simulink model "stateflow6DoF"  (R2024b)
settings: Solver=VariableStepAuto  StartTime=0.0  StopTime=inf  RelTol=1e-6
model workspace (MAT data in the model file):
  Apogee_stop = 0
  BG0 = [0.173648177667  0  -0.984807753012; 0  1  0; 0.984807753012  0  0.173648177667]
  e = 1.55334303427
  ignition_delay = 0
  include_turbulence = 1
  is_sustainer = 1
  launch_delay = 0
  q0 = [0.766044443119 0 0.642787609687 0]
  rocket = MultiStageRocket
  rocket.Name = "Argonia_2_19"
  rocket.stages(1) = Rocket
  rocket.stages(1).Name = "SustainerStage"
  rocket.stages(1).mass_dry = -2
  rocket.stages(1).XCG_dry = 1.653
  rocket.stages(1).MOI_dry = [0.005  0  0; 0  6.179  0; 0  0  6.179]
  rocket.stages(1).LREF = 0.059055
  rocket.stages(1).SREF = 0.0027390706167
  rocket.stages(1).NC_type = "KARMAN"
  rocket.stages(1).NC_length = 0.333375
  rocket.stages(1).NC_diam = 0.059055
  rocket.stages(1).AF1_length = 2.62509
  rocket.stages(1).AF1_diam = 0.059055
  rocket.stages(1).FN1_number = [3 3]
  rocket.stages(1).FN1_type = ["HEX" "HEX"]
  rocket.stages(1).FN1_NACA = ["" ""]
  rocket.stages(1).FN1_root = [0.2794 0.3556]
  rocket.stages(1).FN1_tip = [0.071628 0.071628]
  rocket.stages(1).FN1_height = [0.061214 0.0862076]
  rocket.stages(1).FN1_sweep = [72.6438266558 72.4181028235]
  rocket.stages(1).FN1_edgeRad = [0.000127 0.000127]
  rocket.stages(1).FN1_XLE = [1.497965 2.590165]
  rocket.stages(1).THICKNESS = [0.004064 0.004064]
  rocket.stages(1).ZUPPER = [0.00727272727273 0.00571428571429]
  rocket.stages(1).ZLOWER = [0.00727272727273 0.00571428571429]
  rocket.stages(1).LMAXU = [0.05 0.05]
  rocket.stages(1).LMAXL = [0.05 0.05]
  rocket.stages(1).LFLATU = [0.9 0.9]
  rocket.stages(1).LFLATL = [0.9 0.9]
  rocket.stages(1).m_table = [0.01  8.429; 0.02  8.423; 0.03  8.416; 0.04  8.409; 0.05  8.402; 0.06  8.396; 0.07  8.389; 0.08  8.383; 0.09  8.376; 0.1  8.369; 0.11  8.363; 0.12  8.356; 0.13  8.35; 0.14  8.343; 0.15  8.336; 0.16  8.33; 0.17  8.323; 0.18  8.317; 0.19  8.31; 0.2  8.304; 0.21  8.297; 0.22  8.291; 0.23  8.284; 0.24  8.278; 0.255  8.268; 0.278  8.253; 0.311  8.231; 0.361  8.199; 0.411  8.167; 0.461  8.135; 0.511  8.104; 0.561  8.072; 0.611  8.04; 0.661  8.009; 0.711  7.977; 0.761  7.946; 0.811  7.914; 0.861  7.883; 0.911  7.852; 0.961  7.821; 1.003  7.795; 1.04  7.772; 1.076  7.75; 1.113  7.727; 1.154  7.702; 1.204  7.672; 1.254  7.641; 1.304  7.612; 1.352  7.583; 1.385  7.564; 1.415  7.546; 1.445  7.528; 1.479  7.508; 1.525  7.481; 1.575  7.452; 1.625  7.423; 1.658  7.404; 1.687  7.388; 1.716  7.371; 1.749  7.352; 1.799  7.325; 1.849  7.297; 1.888  7.276; 1.917  7.26; 1.946  7.244; 1.982  7.225; 2.032  7.199; 2.082  7.174; 2.113  7.159; 2.143  7.146; 2.181  7.132; 2.231  7.115; 2.281  7.1; 2.314  7.092; 2.35  7.083; 2.4  7.072; 2.45  7.064; 2.49  7.058; 2.531  7.051; 2.581  7.044; 2.631  7.04; 2.676  7.037; 2.726  7.035; 2.776  7.033; 2.826  7.033; 2.876  7.032; 2.926  7.032; 2.976  7.031; 3  7.031]
  rocket.stages(1).COM_table = [0.01  1.817; 0.02  1.816; 0.03  1.816; 0.04  1.815; 0.05  1.814; 0.06  1.814; 0.07  1.813; 0.08  1.812; 0.09  1.812; 0.1  1.811; 0.11  1.81; 0.12  1.81; 0.13  1.809; 0.14  1.808; 0.15  1.808; 0.16  1.807; 0.17  1.806; 0.18  1.806; 0.19  1.805; 0.2  1.805; 0.21  1.804; 0.22  1.803; 0.23  1.803; 0.24  1.802; 0.255  1.801; 0.278  1.799; 0.311  1.797; 0.361  1.794; 0.411  1.791; 0.461  1.787; 0.511  1.784; 0.561  1.781; 0.611  1.777; 0.661  1.774; 0.711  1.77; 0.761  1.767; 0.811  1.763; 0.861  1.76; 0.911  1.756; 0.961  1.753; 1.003  1.75; 1.04  1.747; 1.076  1.745; 1.113  1.742; 1.154  1.739; 1.204  1.736; 1.254  1.732; 1.304  1.728; 1.352  1.725; 1.385  1.723; 1.415  1.721; 1.445  1.718; 1.479  1.716; 1.525  1.713; 1.575  1.709; 1.625  1.705; 1.658  1.703; 1.687  1.701; 1.716  1.699; 1.749  1.696; 1.799  1.693; 1.849  1.689; 1.888  1.686; 1.917  1.684; 1.946  1.682; 1.982  1.68; 2.032  1.676; 2.082  1.673; 2.113  1.671; 2.143  1.669; 2.181  1.667; 2.231  1.665; 2.281  1.663; 2.314  1.662; 2.35  1.66; 2.4  1.659; 2.45  1.658; 2.49  1.657; 2.531  1.656; 2.581  1.655; 2.631  1.654; 2.676  1.654; 2.726  1.654; 2.776  1.653; 2.826  1.653; 2.876  1.653; 2.926  1.653; 2.976  1.653; 3  1.653]
  rocket.stages(1).MOI_table = [0.006 0.006 0.006 0.006 0.006 0.006 0.006 0.006 0.006 0.006 0.006 0.006 ... (801 elements, 89x3x3)]
  rocket.stages(1).motor = SolidMotor
  rocket.stages(1).motor.Name = "AeroTech HP-L1000W"
  rocket.stages(1).motor.thrust_table = [0.01  332.093; 0.02  1267.419; 0.03  1294.701; 0.04  1313.086; 0.05  1319.183; 0.06  1312.991; 0.07  1306.8; 0.08  1300.608; 0.09  1294.416; 0.1  1288.224; 0.11  1282.033; 0.12  1275.841; 0.13  1269.649; 0.14  1263.457; 0.15  1257.266; 0.16  1251.074; 0.17  1244.882; 0.18  1238.69; 0.19  1232.499; 0.2  1228.068; 0.21  1234.206; 0.22  1242.105; 0.23  1250.004; 0.24  1257.903; 0.255  1266.148; 0.278  1259.177; 0.311  1245.662; 0.361  1247.95; 0.411  1239.736; 0.461  1217.022; 0.511  1219.715; 0.561  1222.613; 0.611  1225.365; 0.661  1224.251; 0.711  1221.415; 0.761  1218.579; 0.811  1215.428; 0.861  1210.092; 0.911  1204.338; 0.961  1198.584; 1.003  1193.301; 1.04  1188.756; 1.076  1184.609; 1.113  1181.332; 1.154  1178.132; 1.204  1174.387; 1.254  1170.286; 1.304  1164.499; 1.352  1156.078; 1.385  1149.076; 1.415  1143.601; 1.445  1138.375; 1.479  1132.822; 1.525  1125.967; 1.575  1118.328; 1.625  1110.52; 1.658  1103.994; 1.687  1099.14; 1.716  1094.669; 1.749  1089.82; 1.799  1079.006; 1.849  1063.36; 1.888  1051.16; 1.917  1048.821; 1.946  1047.63; 1.982  1046.301; 2.032  1026.685; 2.082  960.979; 2.113  897.673; 2.143  821.694; 2.181  741.135; 2.231  659.341; 2.281  569.943; 2.314  513.948; 2.35  472.863; 2.4  421.86; 2.45  364.372; 2.49  313.538; 2.531  267.801; 2.581  216.206; 2.631  165.618; 2.676  121.617; 2.726  80.868; 2.776  49.756; 2.826  35.45; 2.876  26.526; 2.926  17.603; 2.976  8.679; 3  2.109]
  rocket.stages(1).motor.mass_table = [0.01  3.984; 0.02  3.977; 0.03  3.971; 0.04  3.964; 0.05  3.957; 0.06  3.951; 0.07  3.944; 0.08  3.937; 0.09  3.931; 0.1  3.924; 0.11  3.918; 0.12  3.911; 0.13  3.904; 0.14  3.898; 0.15  3.891; 0.16  3.885; 0.17  3.878; 0.18  3.871; 0.19  3.865; 0.2  3.858; 0.21  3.852; 0.22  3.845; 0.23  3.839; 0.24  3.832; 0.255  3.823; 0.278  3.808; 0.311  3.786; 0.361  3.754; 0.411  3.722; 0.461  3.69; 0.511  3.659; 0.561  3.627; 0.611  3.595; 0.661  3.564; 0.711  3.532; 0.761  3.5; 0.811  3.469; 0.861  3.438; 0.911  3.407; 0.961  3.376; 1.003  3.35; 1.04  3.327; 1.076  3.305; 1.113  3.282; 1.154  3.257; 1.204  3.227; 1.254  3.196; 1.304  3.166; 1.352  3.138; 1.385  3.118; 1.415  3.101; 1.445  3.083; 1.479  3.063; 1.525  3.036; 1.575  3.007; 1.625  2.978; 1.658  2.959; 1.687  2.943; 1.716  2.926; 1.749  2.907; 1.799  2.88; 1.849  2.852; 1.888  2.83; 1.917  2.815; 1.946  2.799; 1.982  2.779; 2.032  2.754; 2.082  2.728; 2.113  2.714; 2.143  2.701; 2.181  2.687; 2.231  2.67; 2.281  2.655; 2.314  2.647; 2.35  2.638; 2.4  2.626; 2.45  2.619; 2.49  2.612; 2.531  2.606; 2.581  2.599; 2.631  2.595; 2.676  2.592; 2.726  2.589; 2.776  2.588; 2.826  2.588; 2.876  2.587; 2.926  2.587; 2.976  2.586; 3  2.586]
  rocket.stages(1).motor.dry_mass = 2.586
  rocket.stages(1).motor.total_prop_mass = 1.398
  rocket.stages(1).motor.motor_length = 0.635
  rocket.stages(1).motor.motor_diameter = 0.054
  rocket.stages(2) = Rocket
  rocket.stages(2).Name = "Stage"
  rocket.stages(2).mass_dry = -1
  rocket.stages(2).XCG_dry = 0.659935
  rocket.stages(2).MOI_dry = [0.002  0  0; 0  0.252  0; 0  0  0.252]
  rocket.stages(2).LREF = 0.059055
  rocket.stages(2).SREF = 0.0027390706167
  rocket.stages(2).NC_diam = 0.059055
  rocket.stages(2).AF1_length = 1.1684
  rocket.stages(2).AF1_diam = 0.059055
  rocket.stages(2).FN1_number = 3
  rocket.stages(2).FN1_root = 0.3556
  rocket.stages(2).FN1_tip = 0.071628
  rocket.stages(2).FN1_height = 0.0862076
  rocket.stages(2).FN1_sweep = 72.4181028235
  rocket.stages(2).FN1_XLE = 0.8001
  rocket.stages(2).THICKNESS = 0.004064
  rocket.stages(2).ZUPPER = 0.00571428571429
  rocket.stages(2).ZLOWER = 0.00571428571429
  rocket.stages(2).LMAXU = 0.05
  rocket.stages(2).LMAXL = 0.05
  rocket.stages(2).LFLATU = 0.9
  rocket.stages(2).LFLATL = 0.9
  rocket.stages(2).m_table = [8.022  2.518; 8.055  2.518]
  rocket.stages(2).COM_table = [6.231935  0.659935; 6.264935  0.659935]
  rocket.stages(2).MOI_table = reshape([0.002 0.002 0 0 0 0 0 0 0.252 0.252 0 0 0 0 0 0 0.252 0.252], [2 3 3])
  rocket.stages(2).motor = SolidMotor
  rocket.stages(2).motor.Name = "AeroTech HP-L1000W"
  rocket.stages(2).motor.thrust_table = [0.01  332.093; 0.02  1267.419; 0.03  1294.701; 0.04  1313.086; 0.05  1319.183; 0.06  1312.991; 0.07  1306.8; 0.08  1300.608; 0.09  1294.416; 0.1  1288.224; 0.11  1282.033; 0.12  1275.841; 0.13  1269.649; 0.14  1263.457; 0.15  1257.266; 0.16  1251.074; 0.17  1244.882; 0.18  1238.69; 0.19  1232.499; 0.2  1228.068; 0.21  1234.206; 0.22  1242.105; 0.23  1250.004; 0.24  1257.903; 0.255  1266.148; 0.278  1259.177; 0.311  1245.662; 0.361  1247.95; 0.411  1239.736; 0.461  1217.022; 0.511  1219.715; 0.561  1222.613; 0.611  1225.365; 0.661  1224.251; 0.711  1221.415; 0.761  1218.579; 0.811  1215.428; 0.861  1210.092; 0.911  1204.338; 0.961  1198.584; 1.003  1193.301; 1.04  1188.756; 1.076  1184.609; 1.113  1181.332; 1.154  1178.132; 1.204  1174.387; 1.254  1170.286; 1.304  1164.499; 1.352  1156.078; 1.385  1149.076; 1.415  1143.601; 1.445  1138.375; 1.479  1132.822; 1.525  1125.967; 1.575  1118.328; 1.625  1110.52; 1.658  1103.994; 1.687  1099.14; 1.716  1094.669; 1.749  1089.82; 1.799  1079.006; 1.849  1063.36; 1.888  1051.16; 1.917  1048.821; 1.946  1047.63; 1.982  1046.301; 2.032  1026.685; 2.082  960.979; 2.113  897.673; 2.143  821.694; 2.181  741.135; 2.231  659.341; 2.281  569.943; 2.314  513.948; 2.35  472.863; 2.4  421.86; 2.45  364.372; 2.49  313.538; 2.531  267.801; 2.581  216.206; 2.631  165.618; 2.676  121.617; 2.726  80.868; 2.776  49.756; 2.826  35.45; 2.876  26.526; 2.926  17.603; 2.976  8.679; 3  2.109]
  rocket.stages(2).motor.mass_table = [0.01  3.984; 0.02  3.977; 0.03  3.971; 0.04  3.964; 0.05  3.957; 0.06  3.951; 0.07  3.944; 0.08  3.937; 0.09  3.931; 0.1  3.924; 0.11  3.918; 0.12  3.911; 0.13  3.904; 0.14  3.898; 0.15  3.891; 0.16  3.885; 0.17  3.878; 0.18  3.871; 0.19  3.865; 0.2  3.858; 0.21  3.852; 0.22  3.845; 0.23  3.839; 0.24  3.832; 0.255  3.823; 0.278  3.808; 0.311  3.786; 0.361  3.754; 0.411  3.722; 0.461  3.69; 0.511  3.659; 0.561  3.627; 0.611  3.595; 0.661  3.564; 0.711  3.532; 0.761  3.5; 0.811  3.469; 0.861  3.438; 0.911  3.407; 0.961  3.376; 1.003  3.35; 1.04  3.327; 1.076  3.305; 1.113  3.282; 1.154  3.257; 1.204  3.227; 1.254  3.196; 1.304  3.166; 1.352  3.138; 1.385  3.118; 1.415  3.101; 1.445  3.083; 1.479  3.063; 1.525  3.036; 1.575  3.007; 1.625  2.978; 1.658  2.959; 1.687  2.943; 1.716  2.926; 1.749  2.907; 1.799  2.88; 1.849  2.852; 1.888  2.83; 1.917  2.815; 1.946  2.799; 1.982  2.779; 2.032  2.754; 2.082  2.728; 2.113  2.714; 2.143  2.701; 2.181  2.687; 2.231  2.67; 2.281  2.655; 2.314  2.647; 2.35  2.638; 2.4  2.626; 2.45  2.619; 2.49  2.612; 2.531  2.606; 2.581  2.599; 2.631  2.595; 2.676  2.592; 2.726  2.589; 2.776  2.588; 2.826  2.588; 2.876  2.587; 2.926  2.587; 2.976  2.586; 3  2.586]
  rocket.stages(2).motor.dry_mass = 2.586
  rocket.stages(2).motor.total_prop_mass = 1.398
  rocket.stages(2).motor.motor_length = 0.635
  rocket.stages(2).motor.motor_diameter = 0.054
  rocket.stages(3) = Rocket
  rocket.stages(3).Name = "Sustainer"
  rocket.stages(3).mass_dry = -1
  rocket.stages(3).XCG_dry = 1.099
  rocket.stages(3).MOI_dry = [0.002  0  0; 0  0.967  0; 0  0  0.967]
  rocket.stages(3).LREF = 0.059055
  rocket.stages(3).SREF = 0.0027390706167
  rocket.stages(3).NC_type = "KARMAN"
  rocket.stages(3).NC_length = 0.333375
  rocket.stages(3).NC_diam = 0.059055
  rocket.stages(3).AF1_length = 1.45669
  rocket.stages(3).AF1_diam = 0.059055
  rocket.stages(3).FN1_number = 3
  rocket.stages(3).FN1_root = 0.2794
  rocket.stages(3).FN1_tip = 0.071628
  rocket.stages(3).FN1_height = 0.061214
  rocket.stages(3).FN1_sweep = 72.6438266558
  rocket.stages(3).FN1_XLE = 1.497965
  rocket.stages(3).THICKNESS = 0.004064
  rocket.stages(3).ZUPPER = 0.00727272727273
  rocket.stages(3).ZLOWER = 0.00727272727273
  rocket.stages(3).LMAXU = 0.05
  rocket.stages(3).LMAXL = 0.05
  rocket.stages(3).LFLATU = 0.9
  rocket.stages(3).LFLATL = 0.9
  rocket.stages(3).m_table = [0  7.031; 0.022  4.508; 0.055  4.496; 0.104  4.476; 0.154  4.46; 0.204  4.448; 0.254  4.436; 0.304  4.426; 0.354  4.416; 0.404  4.406; 0.454  4.396; 0.504  4.386; 0.554  4.377; 0.604  4.368; 0.654  4.359; 0.704  4.35; 0.754  4.341; 0.804  4.332; 0.854  4.323; 0.904  4.314; 0.954  4.305; 1.004  4.297; 1.054  4.288; 1.104  4.279; 1.154  4.271; 1.204  4.262; 1.254  4.253; 1.304  4.245; 1.354  4.236; 1.404  4.228; 1.454  4.219; 1.504  4.21; 1.554  4.202; 1.604  4.193; 1.654  4.185; 1.704  4.177; 1.754  4.168; 1.804  4.16; 1.854  4.152; 1.904  4.143; 1.954  4.135; 2.004  4.126; 2.054  4.118; 2.104  4.109; 2.154  4.101; 2.204  4.093; 2.254  4.084; 2.304  4.076; 2.354  4.067; 2.404  4.059; 2.454  4.05; 2.504  4.042; 2.554  4.034; 2.604  4.025; 2.654  4.017; 2.704  4.008; 2.754  4; 2.804  3.992; 2.854  3.983; 2.904  3.975; 2.954  3.966; 3.004  3.958; 3.054  3.95; 3.104  3.942; 3.154  3.933; 3.204  3.925; 3.254  3.917; 3.304  3.909; 3.354  3.901; 3.404  3.893; 3.454  3.884; 3.504  3.876; 3.554  3.869; 3.604  3.861; 3.654  3.854; 3.704  3.846; 3.754  3.839; 3.804  3.831; 3.854  3.824; 3.904  3.816; 3.954  3.809; 4.004  3.801; 4.054  3.794; 4.104  3.788; 4.154  3.781; 4.204  3.775; 4.254  3.768; 4.304  3.761; 4.354  3.755; 4.404  3.748; 4.454  3.742; 4.504  3.735; 4.554  3.729; 4.604  3.723; 4.654  3.718; 4.704  3.712; 4.754  3.706; 4.804  3.7; 4.854  3.695; 4.904  3.689; 4.954  3.683; 5.004  3.678; 5.054  3.673; 5.104  3.668; 5.154  3.663; 5.204  3.659; 5.254  3.654; 5.304  3.649; 5.354  3.645; 5.404  3.64; 5.454  3.635; 5.504  3.631; 5.554  3.627; 5.604  3.623; 5.654  3.62; 5.704  3.616; 5.754  3.612; 5.804  3.609; 5.854  3.605; 5.904  3.601; 5.954  3.598; 6.004  3.594; 6.054  3.592; 6.104  3.589; 6.154  3.587; 6.204  3.584; 6.254  3.582; 6.304  3.579; 6.354  3.577; 6.404  3.574; 6.454  3.572; 6.504  3.569; 6.554  3.568; 6.604  3.568; 6.654  3.567; 6.704  3.566; 6.754  3.565; 6.804  3.564; 6.854  3.563; 6.904  3.562; 6.954  3.562; 7  3.561]
  rocket.stages(3).COM_table = [0  1.653; 0.022  1.208; 0.055  1.207; 0.104  1.205; 0.154  1.203; 0.204  1.202; 0.254  1.201; 0.304  1.2; 0.354  1.199; 0.404  1.198; 0.454  1.197; 0.504  1.197; 0.554  1.196; 0.604  1.195; 0.654  1.194; 0.704  1.193; 0.754  1.192; 0.804  1.191; 0.854  1.19; 0.904  1.19; 0.954  1.189; 1.004  1.188; 1.054  1.187; 1.104  1.186; 1.154  1.185; 1.204  1.184; 1.254  1.183; 1.304  1.183; 1.354  1.182; 1.404  1.181; 1.454  1.18; 1.504  1.179; 1.554  1.178; 1.604  1.177; 1.654  1.176; 1.704  1.175; 1.754  1.175; 1.804  1.174; 1.854  1.173; 1.904  1.172; 1.954  1.171; 2.004  1.17; 2.054  1.169; 2.104  1.168; 2.154  1.167; 2.204  1.166; 2.254  1.165; 2.304  1.165; 2.354  1.164; 2.404  1.163; 2.454  1.162; 2.504  1.161; 2.554  1.16; 2.604  1.159; 2.654  1.158; 2.704  1.157; 2.754  1.156; 2.804  1.155; 2.854  1.154; 2.904  1.153; 2.954  1.152; 3.004  1.151; 3.054  1.15; 3.104  1.149; 3.154  1.148; 3.204  1.147; 3.254  1.146; 3.304  1.145; 3.354  1.144; 3.404  1.143; 3.454  1.142; 3.504  1.141; 3.554  1.14; 3.604  1.139; 3.654  1.139; 3.704  1.138; 3.754  1.137; 3.804  1.136; 3.854  1.135; 3.904  1.134; 3.954  1.133; 4.004  1.132; 4.054  1.131; 4.104  1.13; 4.154  1.129; 4.204  1.129; 4.254  1.128; 4.304  1.127; 4.354  1.126; 4.404  1.125; 4.454  1.124; 4.504  1.123; 4.554  1.123; 4.604  1.122; 4.654  1.121; 4.704  1.12; 4.754  1.12; 4.804  1.119; 4.854  1.118; 4.904  1.117; 4.954  1.116; 5.004  1.116; 5.054  1.115; 5.104  1.114; 5.154  1.114; 5.204  1.113; 5.254  1.112; 5.304  1.112; 5.354  1.111; 5.404  1.11; 5.454  1.11; 5.504  1.109; 5.554  1.109; 5.604  1.108; 5.654  1.108; 5.704  1.107; 5.754  1.107; 5.804  1.106; 5.854  1.106; 5.904  1.105; 5.954  1.105; 6.004  1.104; 6.054  1.104; 6.104  1.103; 6.154  1.103; 6.204  1.103; 6.254  1.102; 6.304  1.102; 6.354  1.102; 6.404  1.101; 6.454  1.101; 6.504  1.1; 6.554  1.1; 6.604  1.1; 6.654  1.1; 6.704  1.1; 6.754  1.1; 6.804  1.1; 6.854  1.1; 6.904  1.099; 6.954  1.099; 7  1.099]
  rocket.stages(3).MOI_table = [0.005 0.003 0.003 0.003 0.003 0.003 0.003 0.003 0.003 0.003 0.003 0.003 ... (1278 elements, 142x3x3)]
  rocket.stages(3).motor = SolidMotor
  rocket.stages(3).motor.Name = "Loki Research K250-LW"
  rocket.stages(3).motor.thrust_table = [0 0.022 0.055 0.104 0.154 0.204 0.254 0.304 0.354 0.404 0.454 0.504 ... (284 elements, 142x2)]
  rocket.stages(3).motor.mass_table = [0  2.586; 0.022  1.787; 0.055  1.775; 0.104  1.754; 0.154  1.739; 0.204  1.726; 0.254  1.715; 0.304  1.705; 0.354  1.694; 0.404  1.684; 0.454  1.674; 0.504  1.665; 0.554  1.655; 0.604  1.646; 0.654  1.637; 0.704  1.628; 0.754  1.619; 0.804  1.611; 0.854  1.602; 0.904  1.593; 0.954  1.584; 1.004  1.575; 1.054  1.566; 1.104  1.558; 1.154  1.549; 1.204  1.54; 1.254  1.532; 1.304  1.523; 1.354  1.515; 1.404  1.506; 1.454  1.497; 1.504  1.489; 1.554  1.48; 1.604  1.472; 1.654  1.464; 1.704  1.455; 1.754  1.447; 1.804  1.438; 1.854  1.43; 1.904  1.422; 1.954  1.413; 2.004  1.405; 2.054  1.396; 2.104  1.388; 2.154  1.379; 2.204  1.371; 2.254  1.363; 2.304  1.354; 2.354  1.346; 2.404  1.337; 2.454  1.329; 2.504  1.32; 2.554  1.312; 2.604  1.304; 2.654  1.295; 2.704  1.287; 2.754  1.278; 2.804  1.27; 2.854  1.262; 2.904  1.253; 2.954  1.245; 3.004  1.236; 3.054  1.228; 3.104  1.22; 3.154  1.212; 3.204  1.204; 3.254  1.196; 3.304  1.187; 3.354  1.179; 3.404  1.171; 3.454  1.163; 3.504  1.155; 3.554  1.147; 3.604  1.14; 3.654  1.132; 3.704  1.125; 3.754  1.117; 3.804  1.11; 3.854  1.102; 3.904  1.094; 3.954  1.087; 4.004  1.079; 4.054  1.073; 4.104  1.066; 4.154  1.06; 4.204  1.053; 4.254  1.046; 4.304  1.04; 4.354  1.033; 4.404  1.027; 4.454  1.02; 4.504  1.013; 4.554  1.008; 4.604  1.002; 4.654  0.996; 4.704  0.99; 4.754  0.985; 4.804  0.979; 4.854  0.973; 4.904  0.967; 4.954  0.962; 5.004  0.956; 5.054  0.951; 5.104  0.947; 5.154  0.942; 5.204  0.937; 5.254  0.932; 5.304  0.928; 5.354  0.923; 5.404  0.918; 5.454  0.914; 5.504  0.909; 5.554  0.905; 5.604  0.902; 5.654  0.898; 5.704  0.894; 5.754  0.891; 5.804  0.887; 5.854  0.883; 5.904  0.88; 5.954  0.876; 6.004  0.872; 6.054  0.87; 6.104  0.867; 6.154  0.865; 6.204  0.863; 6.254  0.86; 6.304  0.858; 6.354  0.855; 6.404  0.853; 6.454  0.85; 6.504  0.848; 6.554  0.847; 6.604  0.846; 6.654  0.845; 6.704  0.844; 6.754  0.843; 6.804  0.843; 6.854  0.842; 6.904  0.841; 6.954  0.84; 7  0.839]
  rocket.stages(3).motor.dry_mass = 0.839
  rocket.stages(3).motor.total_prop_mass = 1.747
  rocket.stages(3).motor.motor_length = 0.499
  rocket.stages(3).motor.motor_diameter = 0.054
  second_ignition_stop = 0
  separation_delay = 5
  vertical_angle_lockout = 25
  wind_direction_table = [0  180; 1  180]
  wind_model_type = "Wind_Table"
  wind_speed_table = [0  7.15; 1  7.15]
values from neighbouring files (symbols this model uses):
  g = 9.81    [initialize_6DoF.m]
  latlong0 = [initial_conditions.lambda0, initial_conditions.mu0]    [initialize_6DoF.m]    (also in rail_output_to_6DoF_initial_conditions.m = deg2rad([launch_site.latitude;                      launch_s)
  v0_NED = GB0*initial_conditions.uvw0_B    [initialize_6DoF.m]
undefined symbols (not defined in the file or in its folder): aerotables, Cd, ChartModeType, deltat, FlightPhase2, HG0, l, launch_elevation, magnitude, mu, rho, S, uvw0_B
libraries: simulink_extras x6, aerolibfltsims x2, aerolibatmos2 x1, sharedtransform x1, aerolibanim x1
settings Model: DataDictionary=CombinedModelDictionary.sldd  Creator=thatf  LastModifiedBy=thatf
settings SolverCC: ZeroCrossAlgorithm=Adaptive
settings DebuggingCC: IgnoredZcDiagnostic=none
settings HardwareCC: ProdBitPerLong=64  ProdHWDeviceType=Intel->x86-64 (Linux 64)
settings SFSimCC: SimCustomHeaderCode=|
  | #include "pressure_altitude.h"
  | #include "flight_estimation.h"
  | #include "data.h"
  | #include "max_m10s.h"
  | #include "i2c/i2c.h"
settings SFSimCC: SimUserSources=|
  | Ccode/pressure_altitude.c
  | Ccode/my_func.c
  | Ccode/flight_estimation.c
  | Ccode/accel_est.c
  | Ccode/vector.c
settings RTWCC: Description=Simulink Desktop Real-Time  SystemTargetFile=sldrt.tlc  TemplateMakefile=sldrt.tmf  RTWCompilerOptimization=on
settings CodeAppCC: MaxIdLength=95
settings SimulinkDesktopRealTimeCC: TargetLibSuffix=_sldrt.a  TargetPreCompLibLocation=C:\Program Files\MATLAB\R2024b\toolbox\sldrt\lib\win64  ParMdlRefBuildCompliant=on

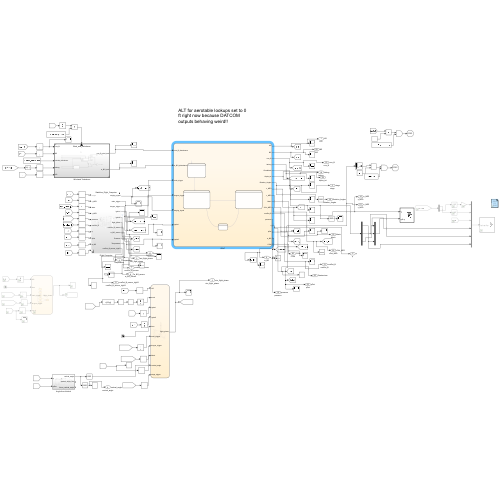
[thumbnail: Simulink's stored preview of the top-level diagram]
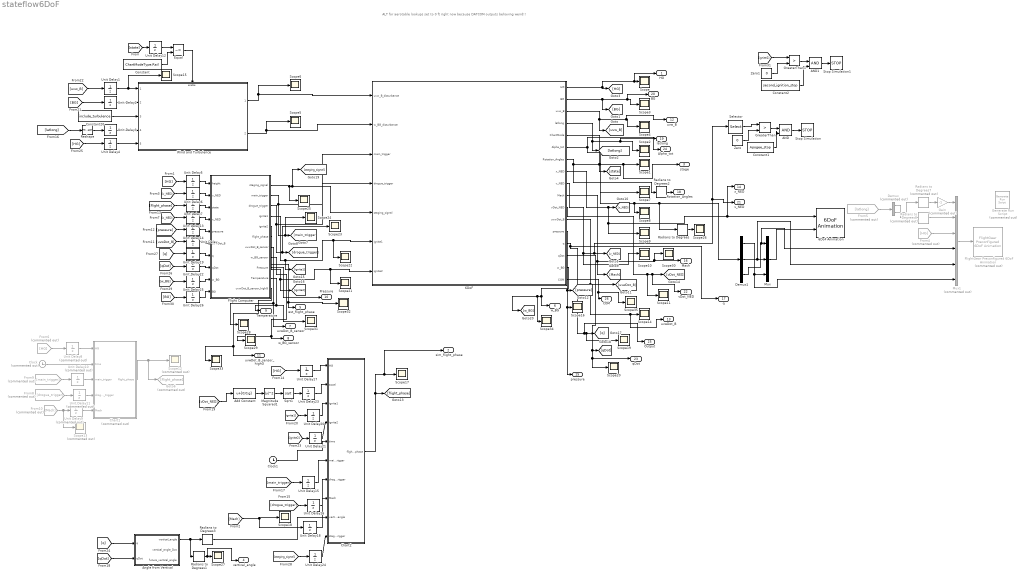
== system stateflow6DoF ==
  note: ALT for aerotable lookups set to 0 ft right now because DATCOM outputs behaving weird!!
  6DoF : Stateflow chart  TreatAsAtomicUnit=on  SystemSampleTime=0
  6DoF Animation : aerolibanim/6DoF Animation  u1=[-10 10 -10 10 -10 10]  u2=0.1  u3=1.0  u4=[0 0 0]  u5=Fly alongside  u6=[8 -8 0]  u7=10  u8=on
  AND : Logic  IconShape=distinctive  AllPortsSameDT=off  OutDataTypeStr=boolean
  AND1 : Logic  IconShape=distinctive  AllPortsSameDT=off  OutDataTypeStr=boolean
  Add Constant : Bias  Bias=[0;0;g]  SaturateOnIntegerOverflow=off
  Angle from Vertical : Subsystem
  Chart1 : Stateflow chart  Commented=on  TreatAsAtomicUnit=on
  Chart2 : Stateflow chart  TreatAsAtomicUnit=on
  Clock : Clock  Commented=on
  Clock1 : Clock
  Constant : Constant  Value=ChartModeType.Rail
  Constant1 : Constant  Value=Apogee_stop
  Constant2 : Constant  Value=second_ignition_stop
  Constant20 : Constant  Value=include_turbulence
  Demux : Demux  Commented=on  Outputs=2
  Demux1 : Demux  Outputs=3
  Equal : RelationalOperator  Operator=~=  OutDataTypeStr=boolean  RndMeth=Simplest  InputSameDT=off
  Flight Computer : Subsystem  Variant=on  VariantChoicesSpecifier={'Flight_Computer', 'Hardware_Flight_Computer', 'Stateflow_Flight_Computer'}  VariantControlMode=label  VariantControl=Flight Computer  LabelModeActiveChoice=Stateflow_Flight_Computer
  FlightGear Preconfigured 6DoF Animation : aerolibfltsims/FlightGear Preconfigured 6DoF Animation  Commented=on  xFlightGearVersion=v2019.1  DestinationIpAddress=127.0.0.1  DestinationPort=5502  SampleTime=1/30  packetVersion=24
  From10 : From  Commented=on  GotoTag=Mach
  From4 : From  Commented=on  GotoTag=HG
  From5 : From  Commented=on  GotoTag=latlong
  From6 : From  Commented=on  GotoTag=HG
  From8 : From  Commented=on  GotoTag=drogue_trigger
  From9 : From  Commented=on  GotoTag=main_trigger
  Gain : Gain  Commented=on  Gain=-1
  Generate Run Script : aerolibfltsims/Generate Run Script  Commented=on  Architecture=Win64  dataFlow=Send  GeometryModelName=SpaceShuttle  AirportId=KSFO  RunwayId=10L  InitialAltitude=HG0  InitialHeading=113  OffsetDistance=4.72  OffsetAzimuth=0  InstallScenery=on  DisableShaders=off  OriginAddress=127.0.0.1  DestinationPort=5502  OriginPort=5505  LocalAddress=127.0.0.1  OutputFileName=runfg.bat  FlightGearBaseDirectory=C:\Program Files\FlightGear 2020.3
  Goto6 : Goto  Commented=on  GotoTag=flight_phase
  GreaterThan : RelationalOperator  Operator=>  OutDataTypeStr=boolean  RndMeth=Simplest  InputSameDT=off
  GreaterThan1 : RelationalOperator  Operator=>  OutDataTypeStr=boolean  RndMeth=Simplest  InputSameDT=off
  Magnitude Squared1 : Math  Operator=magnitude^2
  Mux : Mux  Inputs=3
  Mux1 : Mux  Commented=on  Inputs=6
  Radians to Degrees{,1..3} (4 alike) : simulink_extras/Transformations/Radians to Degrees
  Radians to Degrees7 : simulink_extras/Transformations/Radians to Degrees  Commented=on
  Radians to Degrees8 : simulink_extras/Transformations/Radians to Degrees  Commented=on
  Reshape : Reshape
  Scope{,1..11,14..35} (34 alike) : Scope
  Scope12 : Scope  Commented=on
  Scope13 : Scope  Commented=on
  Selector : Selector  InputPortWidth=3  IndexOptions=Index vector (dialog)  Indices=[3]  OutputSizes=1
  Sqrt1 : Sqrt
  Stop Simulation : Stop
  Stop Simulation1 : Stop
  Unit Delay{,13..16,18,22,24..25} (9 alike) : UnitDelay  SampleTime=-1  HasFrameUpgradeWarning=on
  Unit Delay1 : UnitDelay  InitialCondition=uvw0_B  SampleTime=-1  HasFrameUpgradeWarning=on
  Unit Delay10 : UnitDelay  Commented=on  SampleTime=-1  HasFrameUpgradeWarning=on
  Unit Delay11 : UnitDelay  Commented=on  SampleTime=-1  HasFrameUpgradeWarning=on
  Unit Delay12 : UnitDelay  InitialCondition=ChartModeType.Rail  SampleTime=-1  HasFrameUpgradeWarning=on
  Unit Delay{4..5,17,20..21,23} (6 alike) : UnitDelay  InitialCondition=HG0  SampleTime=-1  HasFrameUpgradeWarning=on
  Unit Delay19 : UnitDelay  InitialCondition=[1;0;0;0]  SampleTime=-1  HasFrameUpgradeWarning=on
  Unit Delay2 : UnitDelay  InitialCondition=BG0  SampleTime=-1  HasFrameUpgradeWarning=on
  Unit Delay26 : UnitDelay  InitialCondition=BG0  SampleTime=-1  HasFrameUpgradeWarning=on
  Unit Delay3 : UnitDelay  InitialCondition=latlong0  SampleTime=-1  HasFrameUpgradeWarning=on
  Unit Delay6 : UnitDelay  InitialCondition=v0_NED  SampleTime=-1  HasFrameUpgradeWarning=on
  Unit Delay7 : UnitDelay  InitialCondition=FlightPhase2.FP_INIT  SampleTime=-1  HasFrameUpgradeWarning=on
  Unit Delay8 : UnitDelay  Commented=on  InitialCondition=HG0  SampleTime=-1  HasFrameUpgradeWarning=on
  Unit Delay9 : UnitDelay  Commented=on  SampleTime=-1  HasFrameUpgradeWarning=on
  Wind and Turbulence : Subsystem  ReferencedSubsystem=Wind_and_Turbulence
  Zero : Constant  Value=0  OutDataTypeStr=Inherit: Inherit via back propagation
  Zero1 : Constant  Value=0  OutDataTypeStr=Inherit: Inherit via back propagation
  HG : Outport  SignalName=HG
  sim_flight_phase : Outport  Port=2  SignalName=sim_flight_phase
  stage : Outport  Port=3  SignalName=stage
  vertical_angle : Outport  Port=4  SignalName=vertical_angle
  est_flight_phase : Outport  Port=5  SignalName=est_flight_phase
  w_BG : Outport  Port=6  SignalName=w_BG
  uvwDot_B_sensor : Outport  Port=7  SignalName=uvwDot_B_sensor
  w_BG_sensor : Outport  Port=8  SignalName=w_BG_sensor
  Temperature : Outport  Port=9  SignalName=Temperature
  Pressure : Outport  Port=10  SignalName=Pressure
  uvwDot_B_sensor_highG : Outport  Port=11  SignalName=uvwDot_B_sensor_highG
  uvw_B : Outport  Port=12  SignalName=uvw_B
  uvwDot_B : Outport  Port=13  SignalName=uvwDot_B
  x_NED : Outport  Port=14  SignalName=x_NED
  pressure : Outport  Port=15  SignalName=pressure
  Mach : Outport  Port=16  SignalName=Mach
  q : Outport  Port=17  SignalName=q
  Rotation_Angles : Outport  Port=18  SignalName=Rotation_Angles
  latlong : Outport  Port=19  SignalName=latlong
  BG : Outport  Port=20  SignalName=BG
  v_NED : Outport  Port=21  SignalName=v_NED
  vDot_NED : Outport  Port=22  SignalName=vDot_NED
  qDot : Outport  Port=23  SignalName=qDot
  Alpha_tot : Outport  Port=24
  Output : Outport  Port=25  SignalName=Quaternions
  COM : Outport  Port=26  SignalName=COM
  wires:
  Constant20/1 -> Wind and Turbulence/3
  6DoF/4(latlong) -> [latlong], latlong/1, Scope2/1
  Wind and Turbulence/1 -> Scope6/1, 6DoF/1(uvw_B_disturbance)
  Wind and Turbulence/2 -> Scope5/1, 6DoF/2(w_BG_disturbance)
  [uvw_B] -> Unit Delay1/1
  Unit Delay1/1 -> Scope15/1, Wind and Turbulence/1
  Unit Delay2/1 -> Wind and Turbulence/2
  [BG] -> Unit Delay2/1
  Unit Delay4/1 -> Wind and Turbulence/5
  Unit Delay3/1 -> Wind and Turbulence/4
  [HG] -> Unit Delay4/1
  [latlong] -> Reshape/1
  Reshape/1 -> Unit Delay3/1
  6DoF/1(HG) -> HG/1, Scope/1, [HG]
  6DoF/2(BG) -> [BG], BG/1, Scope3/1
  6DoF/3(uvw_B) -> [uvw_B], uvw_B/1, Scope4/1
  Constant/1 -> Equal/2
  Equal/1 -> Wind and Turbulence/Enable
  6DoF/6(Alpha_tot) -> Scope7/1, Alpha_tot/1
  Mux/1 -> 6DoF Animation/2
  Demux1/2 -> Mux/2, Mux1/5
  Demux1/3 -> Mux1/4, Mux/1
  Demux1/1 -> Mux/3, Mux1/6
  6DoF/8(x_NED) -> [x_NED], Scope9/1, x_NED/1, 6DoF Animation/1
  [HG] -> Unit Delay5/1
  [v_NED] -> Unit Delay6/1
  6DoF/9(v_NED) -> Scope10/1, v_NED/1, Selector/1, [v_NED]
  [flight_phase] -> Unit Delay7/1
  Radians to Degrees8/1 -> Mux1/2
  Gain/1 -> Mux1/1
  Radians to Degrees7/1 -> Gain/1
  From4/1 -> Mux1/3
  From5/1 -> Demux/1
  Demux/2 -> Radians to Degrees7/1
  Demux/1 -> Radians to Degrees8/1
  Mux1/1 -> FlightGear Preconfigured 6DoF Animation/1
  Unit Delay8/1 -> Chart1/1(HG)
  From6/1 -> Unit Delay8/1
  Chart1/1(flight_phase) -> Goto6/1, Scope12/1
  Clock/1 -> Chart1/2(time)
  From8/1 -> Unit Delay11/1
  Unit Delay11/1 -> Chart1/4(drogue_trigger)
  Unit Delay10/1 -> Chart1/3(main_trigger)
  From9/1 -> Unit Delay10/1
  6DoF/10(Mach) -> [Mach], Mach/1, Scope30/1
  From10/1 -> Scope13/1, Unit Delay9/1
  Unit Delay9/1 -> Chart1/5(Mach)
  6DoF/5(ChartMode) -> [state], stage/1, Scope1/1
  [state] -> Unit Delay12/1
  Unit Delay12/1 -> Equal/1
  6DoF/11(vDot_NED) -> vDot_NED/1, [vDot_NED], Scope11/1
  6DoF/12(uvwDot_B) -> [uvwDot_B], uvwDot_B/1, Scope14/1
  [uvwDot_B] -> Unit Delay/1
  [x_NED] -> Unit Delay13/1
  6DoF/13(pressure) -> pressure/1, Scope16/1, [pressure]
  [pressure] -> Unit Delay14/1
  [drogue_trigger] -> Unit Delay16/1
  [HG] -> Unit Delay17/1
  Unit Delay18/1 -> Chart2/8(Mach)
  [main_trigger] -> Unit Delay15/1
  Clock1/1 -> Chart2/5(time)
  Unit Delay15/1 -> Chart2/6(main_trigger)
  [Mach] -> Scope18/1, Unit Delay18/1
  Chart2/1(flight_phase) -> sim_flight_phase/1, Scope17/1, [flight_phase]
  Unit Delay17/1 -> Chart2/1(HG)
  Unit Delay16/1 -> Chart2/7(drogue_trigger)
  [vDot_NED] -> Add Constant/1
  Add Constant/1 -> Magnitude Squared1/1
  Magnitude Squared1/1 -> Sqrt1/1
  [ignite2] -> Unit Delay21/1
  [ignite1] -> Unit Delay20/1
  Unit Delay20/1 -> Chart2/3(ignite1)
  Unit Delay21/1 -> Chart2/4(ignite2)
  6DoF/14(q) -> Output/1, Scope19/1, [q], q/1
  [q] -> Angle from Vertical/1(q)
  Unit Delay5/1 -> Flight Computer/1(height)
  Unit Delay6/1 -> Flight Computer/2(v_NED)
  Unit Delay7/1 -> Flight Computer/3(state)
  Unit Delay13/1 -> Flight Computer/4(x_NED)
  Unit Delay14/1 -> Flight Computer/5(pressure)
  Unit Delay/1 -> Flight Computer/6(uvwDot_B)
  Flight Computer/1(staging_signal) -> Scope25/1, 6DoF/5(staging_signal), [staging_signal]
  Flight Computer/2(main_trigger) -> Scope24/1, [main_trigger], 6DoF/3(main_trigger)
  Flight Computer/3(drogue_trigger) -> Scope23/1, [drogue_trigger], 6DoF/4(drogue_trigger)
  Flight Computer/4(ignite1) -> [ignite1], Scope22/1, 6DoF/6(ignite1)
  Flight Computer/5(ignite2) -> [ignite2], Scope21/1, 6DoF/7(ignite2)
  [qDot] -> Angle from Vertical/2(qDot)
  6DoF/15(qDot) -> qDot/1, Scope20/1, [qDot]
  Angle from Vertical/1(vertical_angle) -> Radians to Degrees3/1, Radians to Degrees1/1
  [q] -> Unit Delay19/1
  [qDot] -> Unit Delay22/1
  Unit Delay22/1 -> Flight Computer/8(qDot)
  Unit Delay19/1 -> Flight Computer/7(q)
  Sqrt1/1 -> Unit Delay23/1
  Unit Delay23/1 -> Chart2/2(accel)
  6DoF/7(Rotation_Angles) -> Radians to Degrees2/1, Scope8/1, Radians to Degrees/1, Demux1/1
  Radians to Degrees/1 -> Scope26/1
  Radians to Degrees1/1 -> vertical_angle/1, Scope27/1
  Radians to Degrees3/1 -> Chart2/9(vertical_angle)
  Flight Computer/6(flight_phase) -> Scope32/1, est_flight_phase/1
  Zero/1 -> GreaterThan/2
  Selector/1 -> GreaterThan/1
  GreaterThan/1 -> AND/1
  Constant1/1 -> AND/2
  AND/1 -> Stop Simulation/1
  Unit Delay24/1 -> Chart2/10(stage_trigger)
  [staging_signal] -> Unit Delay24/1
  6DoF/16(w_BG) -> Scope34/1, [w_BG], w_BG/1
  [w_BG] -> Unit Delay25/1
  Unit Delay25/1 -> Flight Computer/9(w_BG)
  [BG] -> Unit Delay26/1
  Unit Delay26/1 -> Flight Computer/10(BG)
  Flight Computer/7(uvwDot_B_sensor) -> Scope28/1, uvwDot_B_sensor/1
  Flight Computer/8(w_BG_sensor) -> Scope29/1, w_BG_sensor/1
  Flight Computer/10(Temperature) -> Temperature/1, Scope31/1
  Flight Computer/9(Pressure) -> Pressure/1
  Flight Computer/11(uvwDot_B_sensor_highG) -> Scope33/1, uvwDot_B_sensor_highG/1
  Radians to Degrees2/1 -> Rotation_Angles/1
  GreaterThan1/1 -> AND1/1
  AND1/1 -> Stop Simulation1/1
  Constant2/1 -> AND1/2
  [ignite2] -> GreaterThan1/1
  Zero1/1 -> GreaterThan1/2
  6DoF/17(COM) -> Scope35/1, COM/1

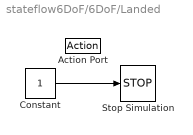
== system stateflow6DoF/6DoF/Landed ==
  Action Port : ActionPort
      settings: CopyFcn=Stateflow.SLINSF.SimulinkMan.removeBlockPreDeleteFcn  PreDeleteFcn=Stateflow.SLINSF.SimulinkMan.unsafePredeleteFcn
  Constant : Constant
  Stop Simulation : Stop
  wires:
  Constant/1 -> Stop Simulation/1

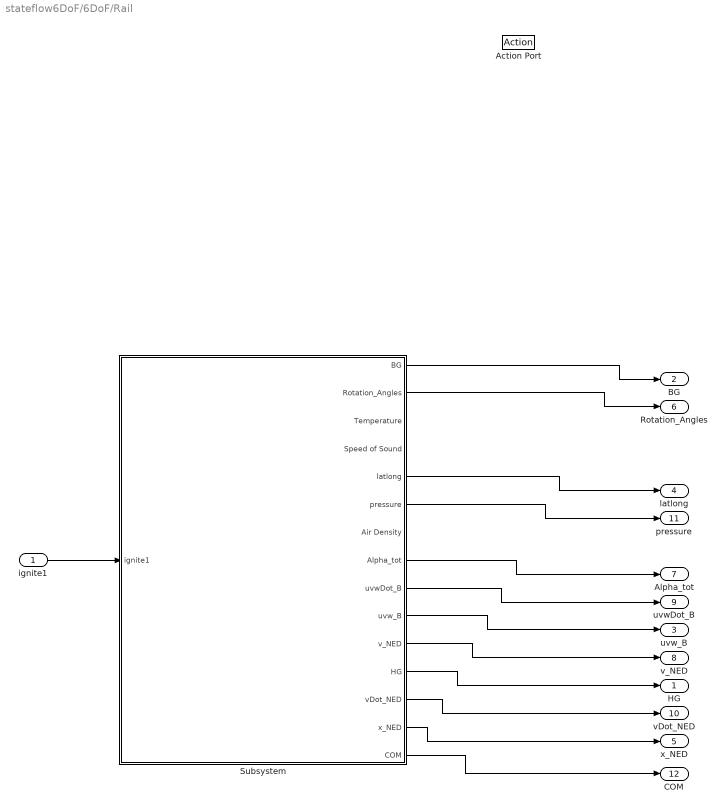
== system stateflow6DoF/6DoF/Rail ==
  ignite1 : Inport
  Action Port : ActionPort
      settings: CopyFcn=Stateflow.SLINSF.SimulinkMan.removeBlockPreDeleteFcn  PreDeleteFcn=Stateflow.SLINSF.SimulinkMan.unsafePredeleteFcn
  Subsystem : Subsystem
  HG : Outport
  BG : Outport  Port=2
  uvw_B : Outport  Port=3
  latlong : Outport  Port=4
  x_NED : Outport  Port=5
  Rotation_Angles : Outport  Port=6
  Alpha_tot : Outport  Port=7
  v_NED : Outport  Port=8
  uvwDot_B : Outport  Port=9
  vDot_NED : Outport  Port=10
  pressure : Outport  Port=11
  COM : Outport  Port=12
  wires:
  Subsystem/1(BG) -> BG/1
  Subsystem/2(Rotation_Angles) -> Rotation_Angles/1
  Subsystem/5(latlong) -> latlong/1
  Subsystem/6(pressure) -> pressure/1
  Subsystem/8(Alpha_tot) -> Alpha_tot/1
  Subsystem/9(uvwDot_B) -> uvwDot_B/1
  Subsystem/10(uvw_B) -> uvw_B/1
  Subsystem/11(v_NED) -> v_NED/1
  Subsystem/12(HG) -> HG/1
  Subsystem/13(vDot_NED) -> vDot_NED/1
  Subsystem/14(x_NED) -> x_NED/1
  ignite1/1 -> Subsystem/1(ignite1)
  Subsystem/15(COM) -> COM/1

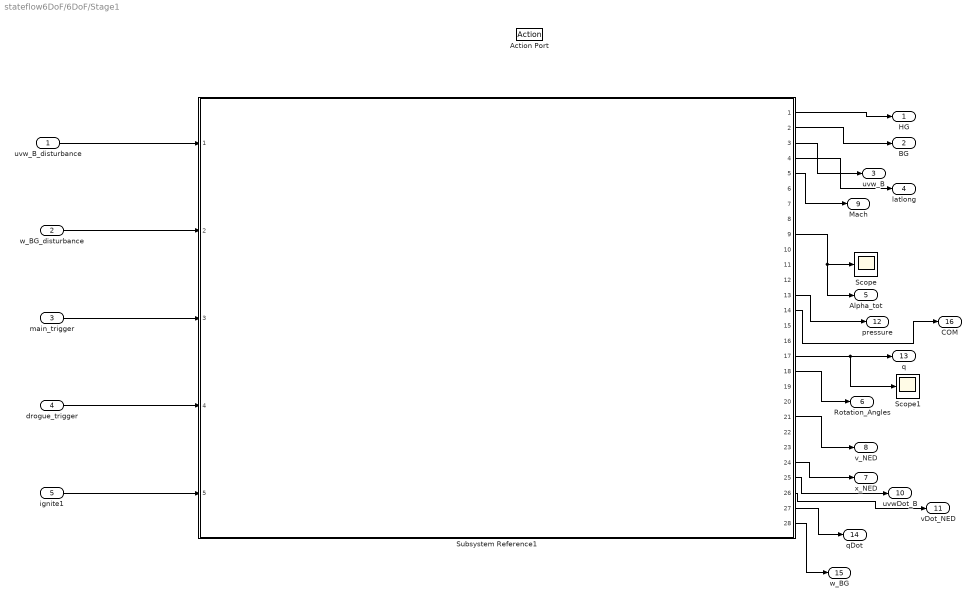
== system stateflow6DoF/6DoF/Stage1 ==
  uvw_B_disturbance : Inport
  w_BG_disturbance : Inport  Port=2
  main_trigger : Inport  Port=3
  drogue_trigger : Inport  Port=4
  ignite1 : Inport  Port=5
  Action Port : ActionPort
      settings: CopyFcn=Stateflow.SLINSF.SimulinkMan.removeBlockPreDeleteFcn  PreDeleteFcn=Stateflow.SLINSF.SimulinkMan.unsafePredeleteFcn
  Scope : Scope
  Scope1 : Scope
  Subsystem Reference1 : Subsystem  ReferencedSubsystem=Copy_of_Shrimple_6dof_parachute  Rocket=rocket.stages(1)  Aerotable=aerotables(1).Aerotable  main_deployment_type=ParachuteDeploymentType.Trigger_Signal_Deployment  drogue_deployment_type=ParachuteDeploymentType.Trigger_Signal_Deployment  time_offset=launch_delay
  HG : Outport
  BG : Outport  Port=2
  uvw_B : Outport  Port=3
  latlong : Outport  Port=4
  Alpha_tot : Outport  Port=5
  Rotation_Angles : Outport  Port=6
  x_NED : Outport  Port=7
  v_NED : Outport  Port=8
  Mach : Outport  Port=9
  uvwDot_B : Outport  Port=10
  vDot_NED : Outport  Port=11
  pressure : Outport  Port=12
  q : Outport  Port=13
  qDot : Outport  Port=14
  w_BG : Outport  Port=15
  COM : Outport  Port=16
  wires:
  Subsystem Reference1/1 -> HG/1
  Subsystem Reference1/2 -> BG/1
  Subsystem Reference1/3 -> uvw_B/1
  Subsystem Reference1/4 -> latlong/1
  drogue_trigger/1 -> Subsystem Reference1/4
  main_trigger/1 -> Subsystem Reference1/3
  Subsystem Reference1/9 -> Alpha_tot/1, Scope/1
  w_BG_disturbance/1 -> Subsystem Reference1/2
  uvw_B_disturbance/1 -> Subsystem Reference1/1
  Subsystem Reference1/17 -> Scope1/1, q/1
  Subsystem Reference1/18 -> Rotation_Angles/1
  Subsystem Reference1/5 -> Mach/1
  Subsystem Reference1/21 -> v_NED/1
  Subsystem Reference1/25 -> uvwDot_B/1
  Subsystem Reference1/26 -> vDot_NED/1
  Subsystem Reference1/13 -> pressure/1
  Subsystem Reference1/27 -> qDot/1
  Subsystem Reference1/28 -> w_BG/1
  Subsystem Reference1/24 -> x_NED/1
  ignite1/1 -> Subsystem Reference1/5
  Subsystem Reference1/14 -> COM/1

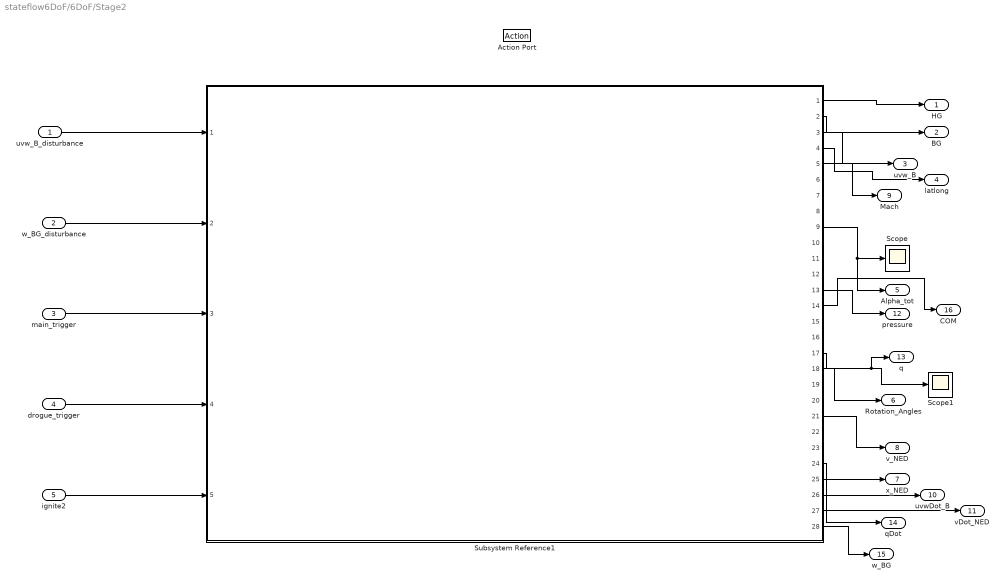
== system stateflow6DoF/6DoF/Stage2 ==
  uvw_B_disturbance : Inport
  w_BG_disturbance : Inport  Port=2
  main_trigger : Inport  Port=3
  drogue_trigger : Inport  Port=4
  ignite2 : Inport  Port=5
  Action Port : ActionPort
      settings: CopyFcn=Stateflow.SLINSF.SimulinkMan.removeBlockPreDeleteFcn  PreDeleteFcn=Stateflow.SLINSF.SimulinkMan.unsafePredeleteFcn
  Scope : Scope
  Scope1 : Scope
  Subsystem Reference1 : Subsystem  ReferencedSubsystem=Copy_of_Shrimple_6dof_parachute  Rocket=rocket.stages(2 + is_sustainer)  Aerotable=aerotables(2 + is_sustainer).Aerotable  main_deployment_type=ParachuteDeploymentType.Trigger_Signal_Deployment  drogue_deployment_type=ParachuteDeploymentType.Trigger_Signal_Deployment  time_offset=0
  HG : Outport
  BG : Outport  Port=2
  uvw_B : Outport  Port=3
  latlong : Outport  Port=4
  Alpha_tot : Outport  Port=5
  Rotation_Angles : Outport  Port=6
  x_NED : Outport  Port=7
  v_NED : Outport  Port=8
  Mach : Outport  Port=9
  uvwDot_B : Outport  Port=10
  vDot_NED : Outport  Port=11
  pressure : Outport  Port=12
  q : Outport  Port=13
  qDot : Outport  Port=14
  w_BG : Outport  Port=15
  COM : Outport  Port=16
  wires:
  Subsystem Reference1/25 -> uvwDot_B/1
  Subsystem Reference1/4 -> latlong/1
  ignite2/1 -> Subsystem Reference1/5
  Subsystem Reference1/21 -> v_NED/1
  Subsystem Reference1/26 -> vDot_NED/1
  Subsystem Reference1/5 -> Mach/1
  drogue_trigger/1 -> Subsystem Reference1/4
  Subsystem Reference1/24 -> x_NED/1
  Subsystem Reference1/1 -> HG/1
  Subsystem Reference1/18 -> Rotation_Angles/1
  uvw_B_disturbance/1 -> Subsystem Reference1/1
  Subsystem Reference1/2 -> BG/1
  main_trigger/1 -> Subsystem Reference1/3
  Subsystem Reference1/3 -> uvw_B/1
  Subsystem Reference1/17 -> q/1, Scope1/1
  w_BG_disturbance/1 -> Subsystem Reference1/2
  Subsystem Reference1/9 -> Alpha_tot/1, Scope/1
  Subsystem Reference1/13 -> pressure/1
  Subsystem Reference1/27 -> qDot/1
  Subsystem Reference1/28 -> w_BG/1
  Subsystem Reference1/14 -> COM/1

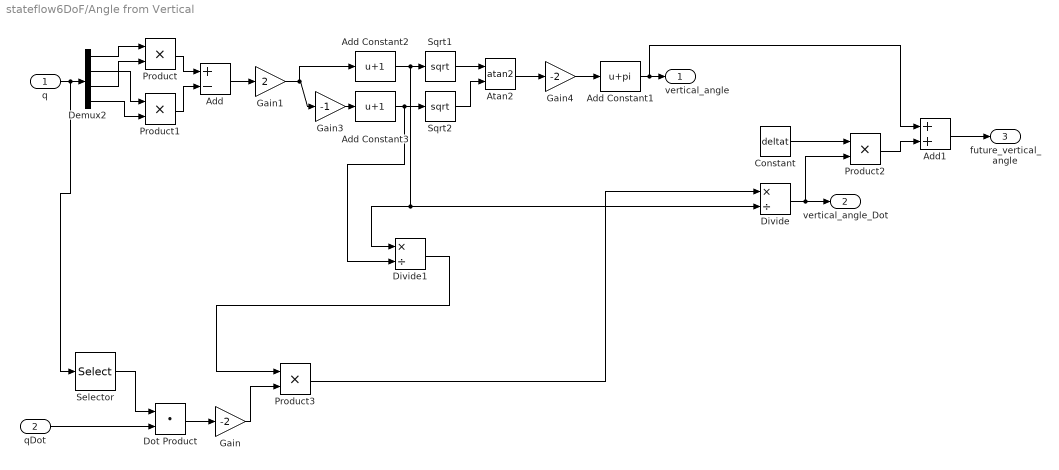
== system stateflow6DoF/Angle from Vertical ==
  q : Inport
  qDot : Inport  Port=2
  Add : Sum  Inputs=+-
  Add Constant1 : Bias  Bias=pi  SaturateOnIntegerOverflow=off
  Add Constant2 : Bias  Bias=1  SaturateOnIntegerOverflow=off
  Add Constant3 : Bias  Bias=1  SaturateOnIntegerOverflow=off
  Add1 : Sum
  Atan2 : Trigonometry  Operator=atan2
  Constant : Constant  Value=deltat
  Demux2 : Demux
  Divide : Product  Inputs=*/
  Divide1 : Product  Inputs=*/
  Dot Product : DotProduct  OutDataTypeStr=Inherit: Inherit via internal rule
  Gain : Gain  Gain=-2
  Gain1 : Gain  Gain=2
  Gain3 : Gain  Gain=-1
  Gain4 : Gain  Gain=-2
  Product{,1..3} (4 alike) : Product
  Selector : Selector  InputPortWidth=4  IndexOptions=Index vector (dialog)  Indices=[3 4 1 2]  OutputSizes=1
  Sqrt1 : Sqrt
  Sqrt2 : Sqrt
  vertical_angle : Outport
  vertical_angle_Dot : Outport  Port=2
  future_vertical_angle : Outport  Port=3
  wires:
  Product/1 -> Add/1
  Demux2/4 -> Product1/2
  Demux2/1 -> Product/1
  Add/1 -> Gain1/1
  Product1/1 -> Add/2
  Demux2/3 -> Product/2
  Demux2/2 -> Product1/1
  q/1 -> Selector/1, Demux2/1
  Selector/1 -> Dot Product/1
  qDot/1 -> Dot Product/2
  Dot Product/1 -> Gain/1
  Divide1/1 -> Product3/1
  Gain/1 -> Product3/2
  Divide/1 -> Product2/2, vertical_angle_Dot/1
  Constant/1 -> Product2/1
  Product2/1 -> Add1/2
  Add1/1 -> future_vertical_angle/1
  Add Constant1/1 -> Add1/1, vertical_angle/1
  Atan2/1 -> Gain4/1
  Gain4/1 -> Add Constant1/1
  Gain3/1 -> Add Constant3/1
  Sqrt1/1 -> Atan2/1
  Sqrt2/1 -> Atan2/2
  Add Constant3/1 -> Divide1/2, Sqrt2/1
  Gain1/1 -> Add Constant2/1, Gain3/1
  Product3/1 -> Divide/1
  Add Constant2/1 -> Divide/2, Divide1/1, Sqrt1/1

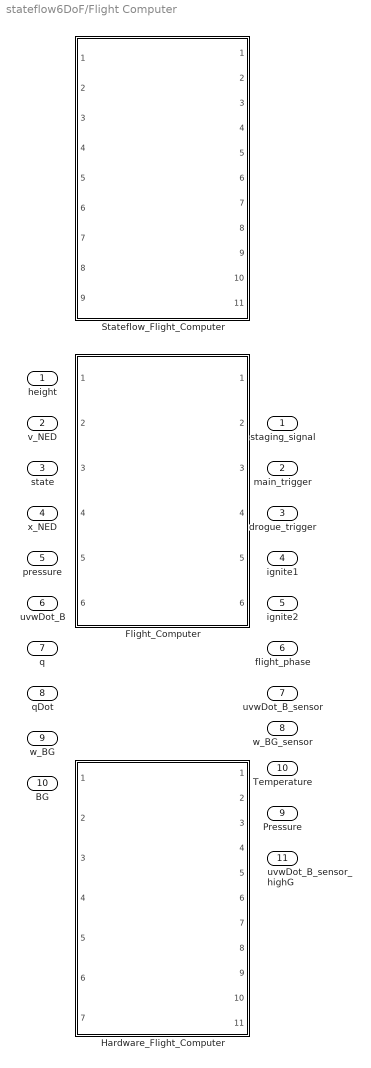
== system stateflow6DoF/Flight Computer ==
  height : Inport
  v_NED : Inport  Port=2
  state : Inport  Port=3
  x_NED : Inport  Port=4
  pressure : Inport  Port=5
  uvwDot_B : Inport  Port=6
  q : Inport  Port=7
  qDot : Inport  Port=8
  w_BG : Inport  Port=9
  BG : Inport  Port=10
  Flight_Computer : Subsystem  VariantControl=Flight_Computer  ReferencedSubsystem=Flight_Computer
  Hardware_Flight_Computer : Subsystem  VariantControl=Hardware_Flight_Computer  ReferencedSubsystem=Hardware_Flight_Computer
  Stateflow_Flight_Computer : Subsystem  VariantControl=Stateflow_Flight_Computer  ReferencedSubsystem=Stateflow_Flight_Computer
  staging_signal : Outport
  main_trigger : Outport  Port=2
  drogue_trigger : Outport  Port=3
  ignite1 : Outport  Port=4
  ignite2 : Outport  Port=5
  flight_phase : Outport  Port=6
  uvwDot_B_sensor : Outport  Port=7
  w_BG_sensor : Outport  Port=8
  Pressure : Outport  Port=9
  Temperature : Outport  Port=10
  uvwDot_B_sensor_highG : Outport  Port=11

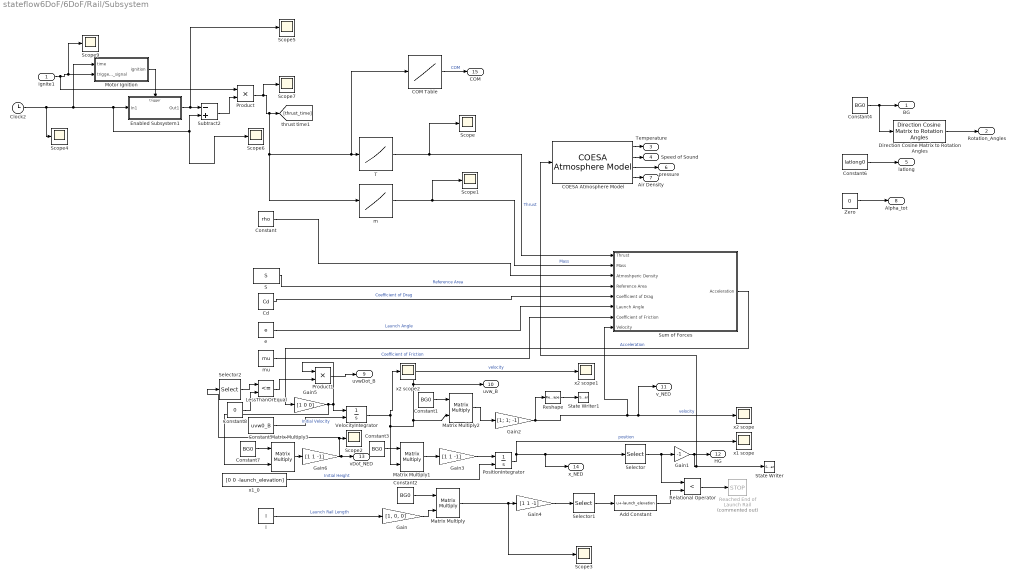
== system stateflow6DoF/6DoF/Rail/Subsystem ==
  ignite1 : Inport
  Add Constant : Bias  Bias=-launch_elevation  SaturateOnIntegerOverflow=off
  COESA Atmosphere Model : aerolibatmos2/COESA Atmosphere Model  units=Metric (MKS)  spec=1976 COESA-extended U.S. Standard Atmosphere  model=Profile  profile_var=High temperature  profile_percent=1%  profile_alt=5 km (16404 ft)  envelope_var=High temperature  envelope_percent=1%  action=Warning
  COM Table : Lookup_n-D  NumberOfTableDimensions=1  BreakpointsForDimension1=rocket.stages(1).COM_table(:,1)  Table=rocket.stages(1).COM_table(:,2)  InternalRulePriority=Speed  RndMeth=Simplest
  Cd : Constant  Value=Cd
  Clock2 : Clock
  Constant : Constant  Value=rho
  Constant{1..4,7} (5 alike) : Constant  Value=BG0
  Constant5 : Constant  Value=uvw0_B
  Constant6 : Constant  Value=latlong0
  Constant8 : Constant  Value=0
  Direction Cosine Matrix to Rotation Angles : sharedtransform/Direction Cosine Matrix to Rotation Angles  rotationOrder=ZYX  aMode=aMode  action=None  tolerance=eps(2)
      settings: LibrarySourceBlock=|
      | aerolibtransform2/Direction Cosine Matrix
      | to Rotation Angles
  Enabled Subsystem1 : Subsystem  TreatAsAtomicUnit=on
  Gain : Gain  Gain=[1, 0, 0]
  Gain1 : Gain  Gain=-1
  Gain2 : Gain  Gain=[1; 1; -1]
  Gain3 : Gain  Gain=[1 1 -1]
  Gain4 : Gain  Gain=[1 1 -1]
  Gain5 : Gain  Gain=[1 0 0]
  Gain6 : Gain  Gain=[1 1 -1]
  LessThanOrEqual : RelationalOperator  Operator=<=  OutDataTypeStr=boolean  RndMeth=Simplest  InputSameDT=off
  Matrix Multiply{,1..3} (4 alike) : Product  Multiplication=Matrix(*)
  Motor Ignition : Subsystem  Variant=on
  PositionIntegrator : Integrator  InitialConditionSource=external  ContinuousStateAttributes='position'
  Product : Product
  Product1 : Product
  Reached End of Launch Rail : Stop  Commented=on
  Relational Operator : RelationalOperator  Operator=<  OutDataTypeStr=boolean  RndMeth=Simplest  InputSameDT=off
  Reshape : Reshape  OutputDimensionality=Column vector (2-D)
  S : Constant  Value=S
  Scope{,1..7,9} (9 alike) : Scope
  Selector : Selector  InputPortWidth=3  IndexOptions=Index vector (dialog)  Indices=[3]  OutputSizes=1
  Selector1 : Selector  InputPortWidth=3  IndexOptions=Index vector (dialog)  Indices=[3]  OutputSizes=1
  Selector2 : Selector  InputPortWidth=3  IndexOptions=Index vector (dialog)  Indices=[3]  OutputSizes=1
  State Writer : StateWriter  StateOwnerBlock=../../../Stage1/Subsystem Reference1/HGIntegrator  StateName=HG
  State Writer1 : StateWriter  StateOwnerBlock=../../../Stage1/Subsystem Reference1/v_NED1  StateName=v_NED
  Subtract2 : Sum  Inputs=-+
  Sum of Forces : Subsystem
  T : Lookup_n-D  NumberOfTableDimensions=1  BreakpointsForDimension1=rocket.stages(1).Tx(:, 1)  Table=rocket.stages(1).Tx(:, 2)  ExtrapMethod=Clip  InternalRulePriority=Speed  RndMeth=Simplest
  VelocityIntegrator : Integrator  InitialConditionSource=external  LimitOutput=on  LowerSaturationLimit=0  ContinuousStateAttributes='uvw_B'
  Zero : Constant  Value=0  OutDataTypeStr=Inherit: Inherit via back propagation
  e : Constant  Value=e
  l : Constant  Value=l
  m : Lookup_n-D  NumberOfTableDimensions=1  BreakpointsForDimension1=rocket.stages(1).m_table(:, 1)  Table=rocket.stages(1).m_table(:, 2)  ExtrapMethod=Clip  UseLastTableValue=on  InternalRulePriority=Speed  RndMeth=Simplest
  mu : Constant  Value=mu
  x1 scope : Scope
  x1_0 : Constant  Value=[0 0 -launch_elevation]
  x2 scope : Scope
  x2 scope1 : Scope
  x2 scope2 : Scope
  BG : Outport
  Rotation_Angles : Outport  Port=2
  Temperature : Outport  Port=3
  Speed of Sound : Outport  Port=4
  latlong : Outport  Port=5
  pressure : Outport  Port=6
  Air Density : Outport  Port=7
  Alpha_tot : Outport  Port=8
  uvwDot_B : Outport  Port=9
  uvw_B : Outport  Port=10
  v_NED : Outport  Port=11
  HG : Outport  Port=12
  vDot_NED : Outport  Port=13
  x_NED : Outport  Port=14
  COM : Outport  Port=15
  wires:
  Matrix Multiply/1 -> Scope3/1, Gain4/1
  Constant2/1 -> Matrix Multiply/1
  Gain5/1 -> Matrix Multiply3/2, Product1/1, VelocityIntegrator/1
  Gain1/1 -> HG/1, State Writer/1, COESA Atmosphere Model/1
  Selector/1 -> Relational Operator/1, Gain1/1
  Constant4/1 -> BG/1, Direction Cosine Matrix to Rotation Angles/1
  mu/1 -> Sum of Forces/7(Coefficient of Friction)  "Coefficient of Friction"
  COESA Atmosphere Model/2 -> Speed of Sound/1
  Constant3/1 -> Matrix Multiply1/1
  COESA Atmosphere Model/3 -> pressure/1
  T/1 -> Scope/1, Sum of Forces/1(Thrust)  "Thrust"
  Cd/1 -> Sum of Forces/5(Coefficient of Drag)  "Coefficient of Drag"
  Zero/1 -> Alpha_tot/1
  PositionIntegrator/1 -> x_NED/1, Selector/1, x1 scope/1  "position"
  l/1 -> Gain/1  "Launch Rail Length"
  S/1 -> Sum of Forces/4(Reference Area)  "Reference Area"
  COESA Atmosphere Model/1 -> Temperature/1
  m/1 -> Scope1/1, Sum of Forces/2(Mass)  "Mass"
  Matrix Multiply3/1 -> Gain6/1
  x1_0/1 -> PositionIntegrator/2  "Initial Height"
  Gain4/1 -> Selector1/1
  Constant1/1 -> Matrix Multiply2/1
  Selector1/1 -> Add Constant/1
  Matrix Multiply1/1 -> Gain3/1
  Sum of Forces/1(" Acceleration") -> Gain5/1  "Acceleration"
  Gain2/1 -> Reshape/1, Sum of Forces/8(Velocity), v_NED/1, x2 scope/1  "velocity"
  Direction Cosine Matrix to Rotation Angles/1 -> Rotation_Angles/1
  Constant7/1 -> Matrix Multiply3/1
  VelocityIntegrator/1 -> x2 scope2/1, uvw_B/1, x2 scope1/1, Matrix Multiply2/2, Matrix Multiply1/2  "velocity"
  e/1 -> Sum of Forces/6(Launch Angle)  "Launch Angle"
  Constant6/1 -> latlong/1
  Add Constant/1 -> Relational Operator/2
  Reshape/1 -> State Writer1/1
  Constant5/1 -> VelocityIntegrator/2  "Initial Velocity"
  Gain6/1 -> Selector2/1, Scope2/1, vDot_NED/1
  Gain/1 -> Matrix Multiply/2
  COESA Atmosphere Model/4 -> Air Density/1
  Constant/1 -> Sum of Forces/3(Atmoshperic Density)
  Gain3/1 -> PositionIntegrator/1
  Matrix Multiply2/1 -> Gain2/1
  Relational Operator/1 -> Reached End of Launch Rail/1
  Subtract2/1 -> Product/2
  Motor Ignition/1(ignition) -> Enabled Subsystem1/Trigger
  ignite1/1 -> Product/1, Scope9/1, Motor Ignition/2(trigger_signal)
  Clock2/1 -> Scope4/1, Motor Ignition/1(time), Enabled Subsystem1/1(In1), Scope6/1, Subtract2/2
  Enabled Subsystem1/1(Out1) -> Scope5/1, Subtract2/1
  Product/1 -> Scope7/1, COM Table/1, T/1, m/1, [thrust_time]
  Product1/1 -> uvwDot_B/1
  LessThanOrEqual/1 -> Product1/2
  Constant8/1 -> LessThanOrEqual/2
  Selector2/1 -> LessThanOrEqual/1
  COM Table/1 -> COM/1  "COM"

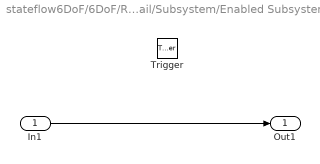
== system stateflow6DoF/6DoF/Rail/Subsystem/Enabled Subsystem1 ==
  In1 : Inport
  Trigger : TriggerPort  VariantControl=(inherit)  InitialTriggerSignalState=zero  PortDimensions=1
  Out1 : Outport
  wires:
  In1/1 -> Out1/1

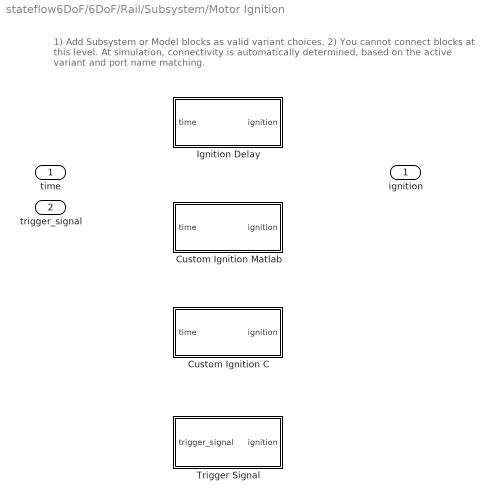
== system stateflow6DoF/6DoF/Rail/Subsystem/Motor Ignition ==
  note: 1) Add Subsystem or Model blocks as valid variant choices.
      | 2) You cannot connect blocks at this level. At simulation, connectivity is automatically
      | determined, based on the active variant and port name matching.
  time : Inport
  trigger_signal : Inport  Port=2
  Custom Ignition C : Subsystem  VariantControl=false
  Custom Ignition Matlab : Subsystem  VariantControl=false
  Ignition Delay : Subsystem  VariantControl=false
  Trigger Signal : Subsystem  VariantControl=true
  ignition : Outport

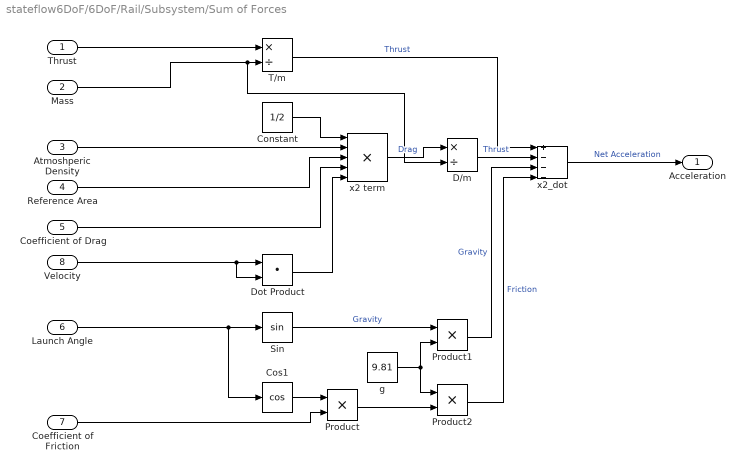
== system stateflow6DoF/6DoF/Rail/Subsystem/Sum of Forces ==
  Thrust : Inport
  Mass : Inport  Port=2
  Atmoshperic Density : Inport  Port=3
  Reference Area : Inport  Port=4
  Coefficient of Drag : Inport  Port=5
  Launch Angle : Inport  Port=6
  Coefficient of Friction : Inport  Port=7
  Velocity : Inport  Port=8
  Constant : Constant  Value=1/2
  Cos1 : Trigonometry  Operator=cos
  D/m : Product  Inputs=*/  RndMeth=Zero  SaturateOnIntegerOverflow=on
  Dot Product : DotProduct  OutDataTypeStr=Inherit: Inherit via internal rule
  Product : Product
  Product1 : Product
  Product2 : Product
  Sin : Trigonometry
  T/m : Product  Inputs=*/  RndMeth=Zero  SaturateOnIntegerOverflow=on
  g : Constant  Value=9.81
  x2 term : Product  Inputs=5
  x2_dot : Sum  Inputs=+---
  " Acceleration" : Outport
  wires:
  Coefficient of Friction/1 -> Product/2
  Sin/1 -> Product1/1  "Gravity"
  Dot Product/1 -> x2 term/5
  Coefficient of Drag/1 -> x2 term/4
  x2 term/1 -> D/m/1  "Drag"
  T/m/1 -> x2_dot/1  "Thrust"
  Atmoshperic Density/1 -> x2 term/2
  Velocity/1 -> Dot Product/2, Dot Product/1
  Launch Angle/1 -> Cos1/1, Sin/1
  Mass/1 -> D/m/2, T/m/2
  Product/1 -> Product2/2
  Cos1/1 -> Product/1
  Reference Area/1 -> x2 term/3
  Thrust/1 -> T/m/1
  x2_dot/1 -> " Acceleration"/1  "Net Acceleration"
  g/1 -> Product1/2, Product2/1
  Product1/1 -> x2_dot/3  "Gravity"
  Product2/1 -> x2_dot/4  "Friction"
  Constant/1 -> x2 term/1
  D/m/1 -> x2_dot/2  "Thrust"

== system stateflow6DoF/6DoF/Rail/Subsystem/Motor Ignition/Custom Ignition C ==
  time : Inport
  ignition : Outport

== system stateflow6DoF/6DoF/Rail/Subsystem/Motor Ignition/Custom Ignition Matlab ==
  time : Inport
  ignition : Outport

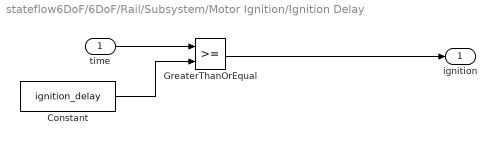
== system stateflow6DoF/6DoF/Rail/Subsystem/Motor Ignition/Ignition Delay ==
  time : Inport
  Constant : Constant  Value=ignition_delay
  GreaterThanOrEqual : RelationalOperator  OutDataTypeStr=boolean  RndMeth=Simplest  InputSameDT=off
  ignition : Outport
  wires:
  time/1 -> GreaterThanOrEqual/1
  Constant/1 -> GreaterThanOrEqual/2
  GreaterThanOrEqual/1 -> ignition/1

== system stateflow6DoF/6DoF/Rail/Subsystem/Motor Ignition/Trigger Signal ==
  trigger_signal : Inport
  ignition : Outport
  wires:
  trigger_signal/1 -> ignition/1

== stateflow chart stateflow6DoF/Chart1 ==
  settings: executeAtInitialization=1
  state FP_BOOST
  state FP_FAST
  state FP_COAST
  state FP_DROGUE
  state FP_LANDED
  state FP_MAIN
  (default) -> FP_BOOST
  FP_BOOST -> FP_FAST : [time > T_end]
  FP_FAST -> FP_COAST : [Mach < 0.8]
  FP_COAST -> FP_LANDED [order 1] : [HG<=launch_elevation]
  FP_COAST -> FP_MAIN [order 3] : [main_trigger == 1]
  FP_COAST -> FP_DROGUE [order 2] : [drogue_trigger == 1]
  FP_DROGUE -> FP_LANDED [order 1] : [HG<=launch_elevation]
  FP_DROGUE -> FP_MAIN [order 2] : [main_trigger == 1]
  FP_MAIN -> FP_LANDED : [HG<=launch_elevation]
  data: T_end constant double =rocket.stages(1).Tx(end,1); HG input; time input; main_trigger input; launch_elevation constant double =launch_elevation; drogue_trigger input; flight_phase output Enum: FlightPhase; Mach input

== stateflow chart stateflow6DoF/Chart2 ==
  settings: executeAtInitialization=1
  state FP_INIT
  state FP_STANDBY
  state FP_PAD
  state FP_IGNITE1
  state FP_BOOST1
  state FP_SEPFAST
  state FP_FAST1
  state FP_SEPCOAST
  state FP_COAST1
  state FP_IGNITE2
  state FP_DROGUE
  state FP_BOOST2
  state FP_MAIN
  state FP_FAST2
  state FP_COAST2
  state FP_LANDED
  (default) -> FP_INIT
  FP_INIT -> FP_STANDBY
  FP_PAD -> FP_STANDBY [order 2] : [vertical_angle >= pad_vertical_angle_lockout]
  FP_STANDBY -> FP_PAD : [vertical_angle < pad_vertical_angle_lockout]
  FP_PAD -> FP_IGNITE1 [order 1] : [ignite1 == 1]
  FP_IGNITE1 -> FP_BOOST1 : [accel>ignite_accel1]
  FP_SEPFAST -> FP_IGNITE2 [order 1] : [ignite2 == 1]
  FP_BOOST1 -> FP_FAST1 : [time > T_end1]
  FP_FAST1 -> FP_SEPFAST [order 3] : [stage_trigger == 1 & is_sus]
  FP_COAST1 -> FP_SEPFAST [order 4] : [stage_trigger == 1 & is_sus]
  FP_SEPFAST -> FP_DROGUE [order 2] : [drogue_trigger == 1]
  FP_SEPFAST -> FP_SEPCOAST [order 4] : [Mach < fast_mach]
  FP_SEPFAST -> FP_MAIN [order 3] : [main_trigger == 1]
  FP_FAST1 -> FP_LANDED [order 1] : [HG<=launch_elevation]
  FP_FAST1 -> FP_COAST1 [order 2] : [Mach < fast_mach]
  FP_SEPCOAST -> FP_IGNITE2 : [ignite2 == 1]
  FP_COAST1 -> FP_LANDED [order 1] : [HG<=launch_elevation]
  FP_COAST1 -> FP_MAIN [order 3] : [main_trigger == 1]
  FP_COAST1 -> FP_DROGUE [order 2] : [drogue_trigger == 1]
  FP_IGNITE2 -> FP_BOOST2 : [accel > ignite_accel2]
  FP_DROGUE -> FP_LANDED [order 1] : [HG<=launch_elevation]
  FP_COAST2 -> FP_DROGUE [order 1] : [drogue_trigger == 1]
  FP_FAST2 -> FP_DROGUE [order 3] : [drogue_trigger == 1]
  FP_DROGUE -> FP_MAIN [order 2] : [main_trigger == 1]
  FP_BOOST2 -> FP_FAST2 : [time > T_end2]
  FP_COAST2 -> FP_MAIN [order 2] : [HG<=launch_elevation]
  FP_FAST2 -> FP_LANDED [order 2] : [HG<=launch_elevation]
  FP_FAST2 -> FP_MAIN [order 4] : [main_trigger == 1]
  FP_MAIN -> FP_LANDED : [HG<=launch_elevation]
  FP_FAST2 -> FP_COAST2 [order 1] : [Mach < 0.8]
  FP_COAST2 -> FP_LANDED [order 3] : [HG <= launch_elevation]
  data: HG input; accel input; ignite1 input; ignite2 input; time input; main_trigger input; launch_elevation constant double =launch_elevation; drogue_trigger input; flight_phase output Enum: FlightPhase2; Mach input; T_end1 constant double =rocket.stages(1).Tx(end,1) + ignition_delay; T_end2 constant double =rocket.stages(3).Tx(end,1) + ignition_delay; fast_mach constant double =0.7; ignite_accel1 constant double; ignite_accel2 constant double; pad_vertical_angle_lockout constant double =15; vertical_angle input; stage_trigger input; is_sus constant double =is_sustainer

== stateflow chart stateflow6DoF/6DoF ==
  settings: updateMethod=CONTINUOUS  sampleTime=0.1
  state Rail
  state Stage1
  state Stage2
  state Landed
  (default) -> Rail
  Rail -> Stage1 : [-BG0(:,1)'*(Rail.position-[0, 0, -launch_elevation])>l]
      | {
      | Stage1.latlong = latlong0
      | Stage1.q = q0'
      | Stage1.w_BN = w0_BN
      | Stage1.uvw_B = Rail.uvw_B
      | Stage1.position = Rail.position
      | }
  Stage1 -> Stage2 [order 1] : [ staging_signal == true]
      | {
      | Stage2.latlong = Stage1.latlong
      | Stage2.position = Stage1.position
      | Stage2.q = Stage1.q
      | Stage2.uvw_B = Stage1.uvw_B
      | Stage2.v_NED = Stage1.v_NED
      | Stage2.w_BN = Stage1.w_BN
      | Stage2.HG = Stage1.HG
      | }
  Stage1 -> Landed [order 2] : [Stage1.HG<=launch_elevation]
  Stage2 -> Landed : [Stage2.HG<=launch_elevation]
  data: sf_internal_action_state_placeholder_data local double size=1 =0; position local; uvw_B local; sf_internal_action_state_placeholder_data local double size=1 =0; position local; latlong local; q local; w_BN local; uvw_B local; v_NED local; HG local; sf_internal_action_state_placeholder_data local double size=1 =0; latlong local; position local; q local; uvw_B local; v_NED local; w_BN local; HG local; sf_internal_action_state_placeholder_data local double size=1 =0; HG output; BG output; BG0 constant double size=[3, 3] =BG0; l constant double =l; launch_elevation constant double =launch_elevation; uvw_B output; latlong output; uvw_B_disturbance input; w_BG_disturbance input; main_trigger input; drogue_trigger input; ChartMode output Enum: ChartModeType; w0_BN constant double size=[3,1] =w0_BN; latlong0 constant double size=[2] =latlong0; q0 constant double size=[1 4] =q0; staging_signal input; Alpha_tot output; Rotation_Angles output; x_NED output; v_NED output; Mach output; vDot_NED output; uvwDot_B output; pressure output; q output =q0'; qDot output =[0;0;0;0]; ignite1 input; ignite2 input; w_BG output; COM output
